simulink model "DroneControl_2018a"  (R2018a)
settings: Solver=VariableStepAuto  StartTime=0.0  StopTime=Tfinal  RelTol=1e-3
values from neighbouring files (symbols this model uses):
  body_rate_0 = [0;0;0]    [SetDroneControl_copy.m]
  Euler_0 = [0;0;0]    [SetDroneControl_copy.m]
  g = [0;0;-9.8]    [SetDroneControl_copy.m]
  I = [[0.1,0,0];[0,0.1,0];[0,0,0.08]]    [SetDroneControl_copy.m]
  m = 0.2    [SetDroneControl_copy.m]
  surround_rate = 0    [SetDroneControl_copy.m]
  ts = 0.01    [SetDroneControl_copy.m]
  XYZ_0 = [1;2;0]    [SetDroneControl_copy.m]
undefined symbols (not defined in the file or in its folder): Xcmd, Ycmd
libraries: simulink x18, vrlib x2, simulink_extras x1
settings Model: NumberOfSteps=10  Creator=blaze8871  LastModifiedBy=blaze8871
settings DataIOCC: SaveTime=off  ReturnWorkspaceOutputs=on
settings SFSimCC: SimUseLocalCustomCode=on
settings RTWCC: RTWUseLocalCustomCode=on

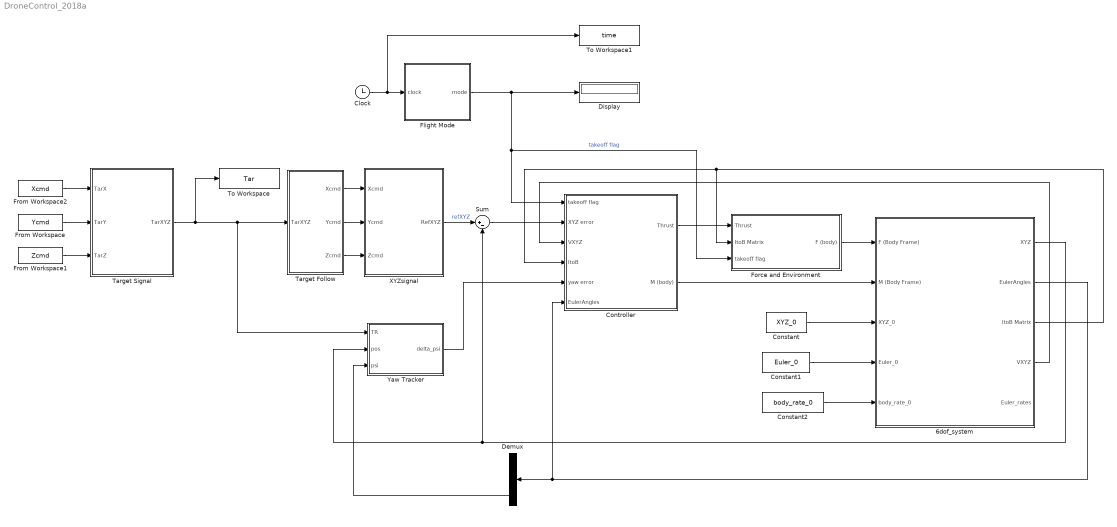
== system DroneControl_2018a ==
  6dof_system : Subsystem
  Clock : Clock
  Constant : Constant  Value=XYZ_0  SampleTime=0.01
  Constant1 : Constant  Value=Euler_0  SampleTime=0.01
  Constant2 : Constant  Value=body_rate_0  SampleTime=0.01
  Controller : Subsystem
  Demux : Demux  Outputs=3
  Display : Display
  Flight Mode : MATLAB Function  TreatAsAtomicUnit=on
  Force and Environment : Subsystem
  From Workspace : FromWorkspace  VariableName=Ycmd  SampleTime=ts
  From Workspace1 : FromWorkspace  VariableName=Zcmd  SampleTime=ts
  From Workspace2 : FromWorkspace  VariableName=Xcmd  SampleTime=ts
  Sum : Sum  Inputs=|+-
  Target Follow : Subsystem
  Target Signal : MATLAB Function  TreatAsAtomicUnit=on
  To Workspace : ToWorkspace  VariableName=Tar  SampleTime=ts
  To Workspace1 : ToWorkspace  VariableName=time  SampleTime=ts
  XYZsignal : MATLAB Function  TreatAsAtomicUnit=on
  Yaw Tracker : MATLAB Function  TreatAsAtomicUnit=on
  wires:
  Constant/1 -> 6dof_system/3(XYZ_0)
  Constant1/1 -> 6dof_system/4(Euler_0)
  Constant2/1 -> 6dof_system/5(body_rate_0)
  6dof_system/3(ItoB Matrix) -> Force and Environment/2(ItoB Matrix), Controller/4(ItoB)
  XYZsignal/1(RefXYZ) -> Sum/1  "refXYZ"
  6dof_system/1(XYZ) -> Sum/2, Yaw Tracker/2(pos)
  Clock/1 -> To Workspace1/1, Flight Mode/1(clock)
  Flight Mode/1(mode) -> Controller/1(takeoff flag), Force and Environment/3(takeoff flag), Display/1  "takeoff flag"
  Force and Environment/1(F (body)) -> 6dof_system/1(F (Body Frame))
  6dof_system/2(EulerAngles) -> Controller/6(EulerAngles), Demux/1
  Sum/1 -> Controller/2(XYZ error)
  6dof_system/4(VXYZ) -> Controller/3(VXYZ)
  Controller/2(M (body)) -> 6dof_system/2(M (Body Frame))
  Controller/1(Thrust) -> Force and Environment/1(Thrust)
  Demux/3 -> Yaw Tracker/3(psi)
  Yaw Tracker/1(delta_psi) -> Controller/5(yaw error)
  Target Signal/1(TarXYZ) -> To Workspace/1, Target Follow/1(TarXYZ), Yaw Tracker/1(TR)
  From Workspace2/1 -> Target Signal/1(TarX)
  From Workspace/1 -> Target Signal/2(TarY)
  From Workspace1/1 -> Target Signal/3(TarZ)
  Target Follow/1(Xcmd) -> XYZsignal/1(Xcmd)
  Target Follow/2(Ycmd) -> XYZsignal/2(Ycmd)
  Target Follow/3(Zcmd) -> XYZsignal/3(Zcmd)

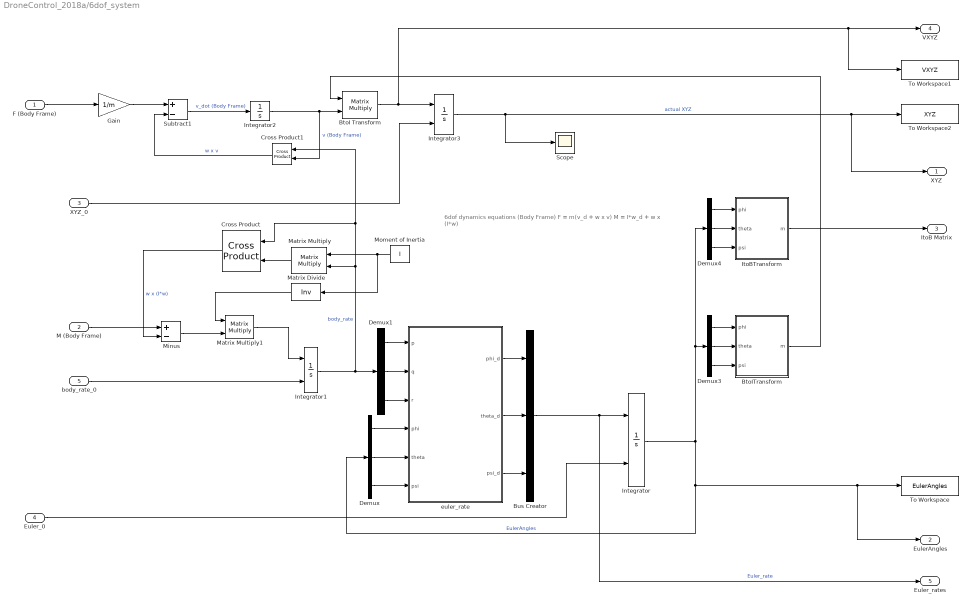
== system DroneControl_2018a/6dof_system ==
  note: 6dof dynamics equations
      | (Body Frame)
      |
      | F = m(v_d + w x v)
      | M = I*w_d + w x (I*w)
  F (Body Frame) : Inport
  M (Body Frame) : Inport  Port=2
  XYZ_0 : Inport  Port=3
  Euler_0 : Inport  Port=4
  body_rate_0 : Inport  Port=5
  BtoI Transform : Product  Multiplication=Matrix(*)
  BtoITransform : MATLAB Function  TreatAsAtomicUnit=on
  Bus Creator : BusCreator  Inputs=3
  Cross Product : vrlib/Utilities/Cross Product
  Cross Product1 : vrlib/Utilities/Cross Product
  Demux{,1,3..4} (4 alike) : Demux  Outputs=3
  Gain : Gain  Gain=1/m
  Integrator : Integrator  InitialConditionSource=external  ContinuousStateAttributes='EulerAngle'
  Integrator1 : Integrator  InitialConditionSource=external  ContinuousStateAttributes='EulerAngle'
  Integrator2 : Integrator
  Integrator3 : Integrator  InitialConditionSource=external
  ItoBTransform : MATLAB Function  TreatAsAtomicUnit=on
  Matrix Divide : Product  Inputs=/  Multiplication=Matrix(*)
  Matrix Multiply : Product  Multiplication=Matrix(*)
  Matrix Multiply1 : Product  Multiplication=Matrix(*)
  Minus : Sum  Inputs=+-
  Moment of Inertia : Constant  Value=I
  Scope : Scope
  Subtract1 : Sum  Inputs=+-
  To Workspace : ToWorkspace  VariableName=EulerAngles  SampleTime=ts
  To Workspace1 : ToWorkspace  VariableName=VXYZ  SampleTime=ts
  To Workspace2 : ToWorkspace  VariableName=XYZ  SampleTime=ts
  euler_rate : MATLAB Function  TreatAsAtomicUnit=on
  XYZ : Outport
  EulerAngles : Outport  Port=2
  ItoB Matrix : Outport  Port=3
  VXYZ : Outport  Port=4
  Euler_rates : Outport  Port=5
  wires:
  F (Body Frame)/1 -> Gain/1
  Demux4/2 -> ItoBTransform/2(theta)
  euler_rate/1(phi_d) -> Bus Creator/1
  BtoITransform/1(m) -> BtoI Transform/1
  Bus Creator/1 -> Euler_rates/1, Integrator/1  "Euler_rate"
  Matrix Multiply/1 -> Cross Product/2
  Moment of Inertia/1 -> Matrix Divide/1, Matrix Multiply/1
  Demux3/2 -> BtoITransform/2(theta)
  Demux/2 -> euler_rate/5(theta)
  Demux4/1 -> ItoBTransform/1(phi)
  Subtract1/1 -> Integrator2/1  "v_dot (Body Frame)"
  Cross Product1/1 -> Subtract1/2  "w x v"
  Demux1/1 -> euler_rate/1(p)
  Demux/3 -> euler_rate/6(psi)
  euler_rate/2(theta_d) -> Bus Creator/2
  Euler_0/1 -> Integrator/2
  Integrator3/1 -> XYZ/1, To Workspace2/1, Scope/1  "actual XYZ"
  Cross Product/1 -> Minus/2  "w x (I*w)"
  M (Body Frame)/1 -> Minus/1
  body_rate_0/1 -> Integrator1/2
  Demux3/3 -> BtoITransform/3(psi)
  euler_rate/3(psi_d) -> Bus Creator/3
  Demux4/3 -> ItoBTransform/3(psi)
  Gain/1 -> Subtract1/1
  Demux3/1 -> BtoITransform/1(phi)
  Demux1/3 -> euler_rate/3(r)
  XYZ_0/1 -> Integrator3/2
  Integrator/1 -> EulerAngles/1, To Workspace/1, Demux/1, Demux4/1, Demux3/1  "EulerAngles"
  Demux/1 -> euler_rate/4(phi)
  Integrator2/1 -> BtoI Transform/2, Cross Product1/2  "v (Body Frame)"
  Integrator1/1 -> Cross Product1/1, Cross Product/1, Matrix Multiply/2, Demux1/1  "body_rate"
  Demux1/2 -> euler_rate/2(q)
  ItoBTransform/1(m) -> ItoB Matrix/1
  BtoI Transform/1 -> To Workspace1/1, VXYZ/1, Integrator3/1
  Minus/1 -> Matrix Multiply1/2
  Matrix Multiply1/1 -> Integrator1/1
  Matrix Divide/1 -> Matrix Multiply1/1

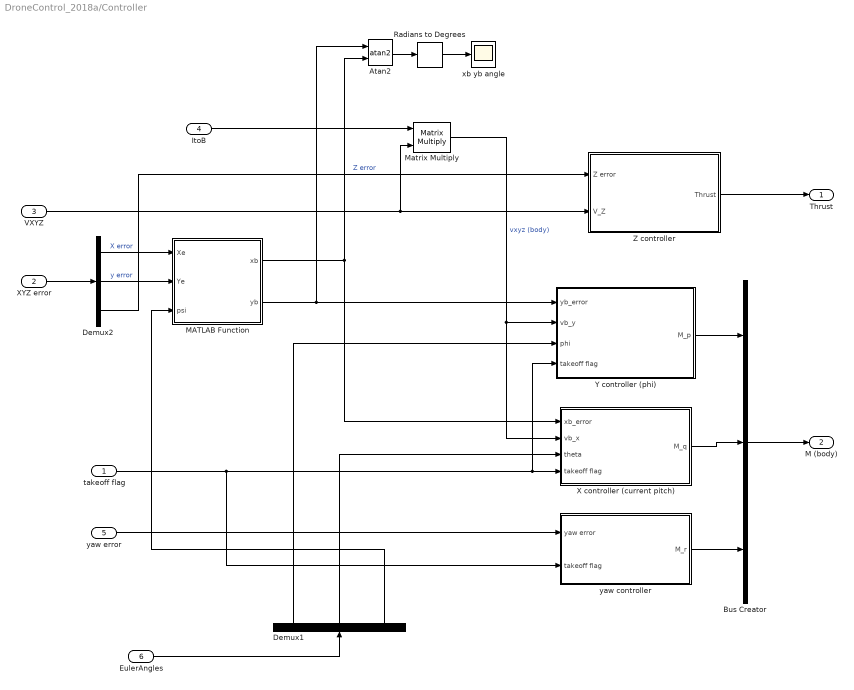
== system DroneControl_2018a/Controller ==
  takeoff flag : Inport
  XYZ error : Inport  Port=2
  VXYZ : Inport  Port=3
  ItoB : Inport  Port=4
  yaw error : Inport  Port=5
  EulerAngles : Inport  Port=6
  Atan2 : Trigonometry  Operator=atan2
  Bus Creator : BusCreator  Inputs=3
  Demux1 : Demux  Outputs=3
  Demux2 : Demux  Outputs=3
  MATLAB Function : MATLAB Function  TreatAsAtomicUnit=on
  Matrix Multiply : Product  Multiplication=Matrix(*)
  Radians to Degrees : simulink_extras/Transformations/Radians to Degrees
  X controller (current pitch) : Subsystem
  Y controller (phi) : Subsystem
  Z controller : Subsystem
  xb yb angle : Scope
  "yaw controller " : Subsystem
  Thrust : Outport
  M (body) : Outport  Port=2
  wires:
  Bus Creator/1 -> M (body)/1
  VXYZ/1 -> Z controller/2(V_Z), Matrix Multiply/2
  "yaw controller "/1(M_r) -> Bus Creator/3
  XYZ error/1 -> Demux2/1
  Demux1/1 -> Y controller (phi)/3(phi)
  Demux1/2 -> X controller (current pitch)/3(theta)
  Demux2/3 -> Z controller/1(Z error)  "Z error"
  takeoff flag/1 -> Y controller (phi)/4(takeoff flag), X controller (current pitch)/4(takeoff flag), "yaw controller "/2(takeoff flag)
  EulerAngles/1 -> Demux1/1
  Y controller (phi)/1(M_p) -> Bus Creator/1
  Demux1/3 -> MATLAB Function/3(psi)
  Z controller/1(Thrust) -> Thrust/1
  Demux2/2 -> MATLAB Function/2(Ye)  "y error"
  yaw error/1 -> "yaw controller "/1(yaw error)
  Demux2/1 -> MATLAB Function/1(Xe)  "X error"
  X controller (current pitch)/1(M_q) -> Bus Creator/2
  MATLAB Function/1(xb) -> X controller (current pitch)/1("xb_error "), Atan2/2
  MATLAB Function/2(yb) -> Atan2/1, Y controller (phi)/1("yb_error ")
  Atan2/1 -> Radians to Degrees/1
  Radians to Degrees/1 -> xb yb angle/1
  ItoB/1 -> Matrix Multiply/1
  Matrix Multiply/1 -> X controller (current pitch)/2(vb_x), Y controller (phi)/2(vb_y)  "vxyz (body)"

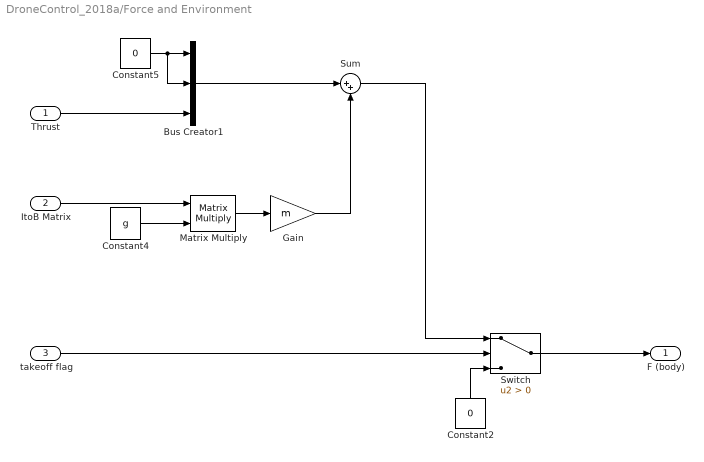
== system DroneControl_2018a/Force and Environment ==
  Thrust : Inport
  ItoB Matrix : Inport  Port=2
  takeoff flag : Inport  Port=3
  Bus Creator1 : BusCreator  Inputs=3
  Constant2 : Constant  Value=0  SampleTime=0.01
  Constant4 : Constant  Value=g  SampleTime=0.01
  Constant5 : Constant  Value=0  SampleTime=0.01
  Gain : Gain  Gain=m
  Matrix Multiply : Product  Multiplication=Matrix(*)
  Sum : Sum  Inputs=|++
  Switch : Switch  Criteria=u2 > Threshold
  F (body) : Outport
  wires:
  Thrust/1 -> Bus Creator1/3
  Bus Creator1/1 -> Sum/1
  Constant4/1 -> Matrix Multiply/2
  ItoB Matrix/1 -> Matrix Multiply/1
  Constant5/1 -> Bus Creator1/2, Bus Creator1/1
  takeoff flag/1 -> Switch/2
  Constant2/1 -> Switch/3
  Matrix Multiply/1 -> Gain/1
  Sum/1 -> Switch/1
  Switch/1 -> F (body)/1
  Gain/1 -> Sum/2

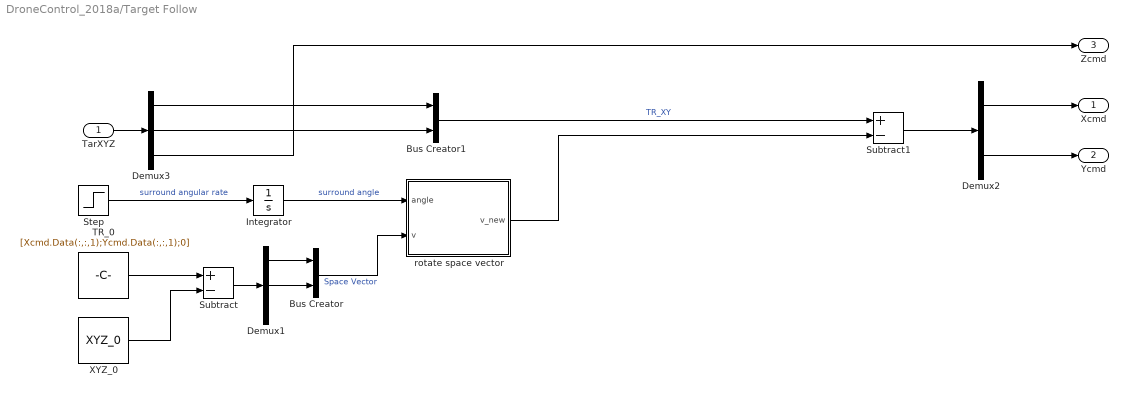
== system DroneControl_2018a/Target Follow ==
  TarXYZ : Inport
  Bus Creator : BusCreator  Inputs=2
  Bus Creator1 : BusCreator  Inputs=2
  Demux1 : Demux  Outputs=3
  Demux2 : Demux  Outputs=2
  Demux3 : Demux  Outputs=3
  Integrator : Integrator
  Step : Step  Time=2  After=surround_rate  SampleTime=0
  Subtract : Sum  Inputs=+-
  Subtract1 : Sum  Inputs=+-
  TR_0 : Constant  Value=[Xcmd.Data(:,:,1);Ycmd.Data(:,:,1);0]
  XYZ_0 : Constant  Value=XYZ_0
  rotate space vector : MATLAB Function  TreatAsAtomicUnit=on
  Xcmd : Outport
  Ycmd : Outport  Port=2
  Zcmd : Outport  Port=3
  wires:
  Subtract1/1 -> Demux2/1
  Demux2/2 -> Ycmd/1
  TR_0/1 -> Subtract/1
  Demux1/2 -> Bus Creator/2
  Bus Creator1/1 -> Subtract1/1  "TR_XY"
  TarXYZ/1 -> Demux3/1
  Demux3/2 -> Bus Creator1/2
  Subtract/1 -> Demux1/1
  Demux3/3 -> Zcmd/1
  Demux2/1 -> Xcmd/1
  Demux1/1 -> Bus Creator/1
  Demux3/1 -> Bus Creator1/1
  Bus Creator/1 -> rotate space vector/2(v)  "Space Vector"
  XYZ_0/1 -> Subtract/2
  Step/1 -> Integrator/1  "surround angular rate"
  Integrator/1 -> rotate space vector/1(angle)  "surround angle"
  rotate space vector/1(v_new) -> Subtract1/2

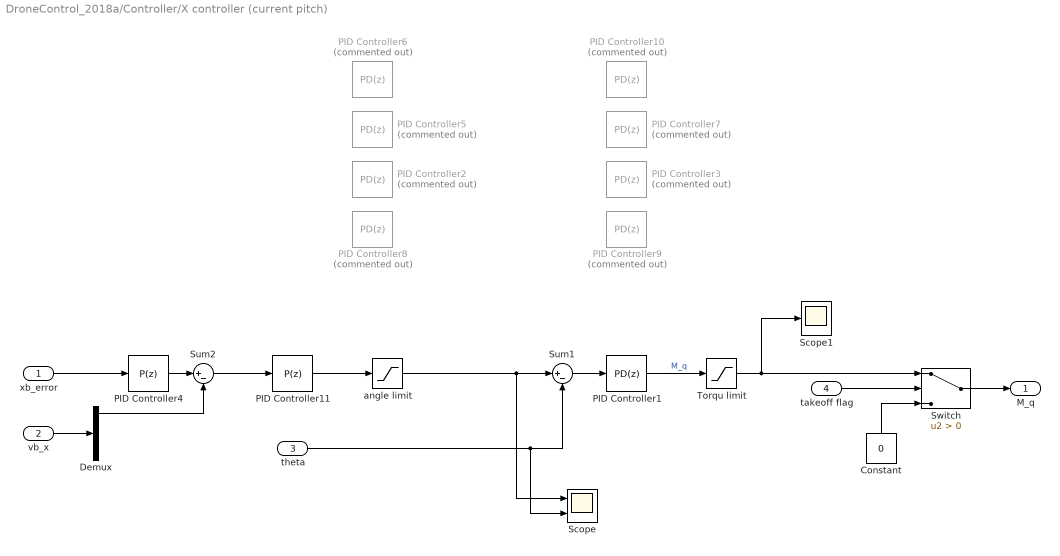
== system DroneControl_2018a/Controller/X controller (current pitch) ==
  "xb_error " : Inport
  vb_x : Inport  Port=2
  theta : Inport  Port=3
  takeoff flag : Inport  Port=4
  Constant : Constant  Value=0
  Demux : Demux  Outputs=3
  PID Controller1 : simulink/Continuous/PID Controller  Controller=PD  Form=Parallel  TimeDomain=Discrete-time  SampleTime=ts  IntegratorMethod=Forward Euler  FilterMethod=Forward Euler  ControllerParametersSource=internal  P=1.1  I=1  D=1.2  UseFilter=on  N=100  TunerSelectOption=Transfer Function Based (PID Tuner App)  InitialConditionSource=internal  InitialConditionForIntegrator=0  InitialConditionForFilter=0  DifferentiatorICPrevScaledInput=0  ExternalReset=none  TrackingMode=off  Kt=1  LimitOutput=off  UpperSaturationLimit=inf  LowerSaturationLimit=-inf  LinearizeAsGain=on  AntiWindupMode=none  Kb=1  POutMin=[]  POutMax=[]  IOutMin=[]  IOutMax=[]  DOutMin=[]  DOutMax=[]  NOutMin=[]  NOutMax=[]  SumOutMin=[]  SumOutMax=[]  SaturationOutMin=[]  SaturationOutMax=[]  PParamMin=[]  PParamMax=[]  IParamMin=[]  IParamMax=[]  DParamMin=[]  DParamMax=[]  NParamMin=[]  NParamMax=[]  KbParamMin=[]  KbParamMax=[]  KtParamMin=[]  KtParamMax=[]  KbOutMin=[]  KbOutMax=[]  KtOutMin=[]  KtOutMax=[]  IntegratorOutMin=[]  IntegratorOutMax=[]  FilterOutMin=[]  FilterOutMax=[]  SumI1OutMin=[]  SumI1OutMax=[]  SumI2OutMin=[]  SumI2OutMax=[]  SumI3OutMin=[]  SumI3OutMax=[]  SumDOutMin=[]  SumDOutMax=[]  DifferentiatorOutMin=[]  DifferentiatorOutMax=[]  FilterDiffOutCoefMin=[]  FilterDiffOutCoefMax=[]  ReciprocalOutMin=[]  ReciprocalOutMax=[]  SumDenOutMin=[]  SumDenOutMax=[]  SumNumOutMin=[]  SumNumOutMax=[]  DivideOutMin=[]  DivideOutMax=[]  IntegratorContinuousStateAttributes=''  IntegratorStateMustResolveToSignalObject=off  IntegratorRTWStateStorageClass=Auto  FilterContinuousStateAttributes=''  FilterStateMustResolveToSignalObject=off  FilterRTWStateStorageClass=Auto
  PID Controller10 : simulink/Continuous/PID Controller  Commented=on  Controller=PD  Form=Parallel  TimeDomain=Discrete-time  SampleTime=ts  IntegratorMethod=Forward Euler  FilterMethod=Forward Euler  ControllerParametersSource=internal  P=0.8  I=1  D=0.5  UseFilter=on  N=100  TunerSelectOption=Transfer Function Based (PID Tuner App)  InitialConditionSource=internal  InitialConditionForIntegrator=0  InitialConditionForFilter=0  DifferentiatorICPrevScaledInput=0  ExternalReset=none  TrackingMode=off  Kt=1  LimitOutput=off  UpperSaturationLimit=inf  LowerSaturationLimit=-inf  LinearizeAsGain=on  AntiWindupMode=none  Kb=1  POutMin=[]  POutMax=[]  IOutMin=[]  IOutMax=[]  DOutMin=[]  DOutMax=[]  NOutMin=[]  NOutMax=[]  SumOutMin=[]  SumOutMax=[]  SaturationOutMin=[]  SaturationOutMax=[]  PParamMin=[]  PParamMax=[]  IParamMin=[]  IParamMax=[]  DParamMin=[]  DParamMax=[]  NParamMin=[]  NParamMax=[]  KbParamMin=[]  KbParamMax=[]  KtParamMin=[]  KtParamMax=[]  KbOutMin=[]  KbOutMax=[]  KtOutMin=[]  KtOutMax=[]  IntegratorOutMin=[]  IntegratorOutMax=[]  FilterOutMin=[]  FilterOutMax=[]  SumI1OutMin=[]  SumI1OutMax=[]  SumI2OutMin=[]  SumI2OutMax=[]  SumI3OutMin=[]  SumI3OutMax=[]  SumDOutMin=[]  SumDOutMax=[]  DifferentiatorOutMin=[]  DifferentiatorOutMax=[]  FilterDiffOutCoefMin=[]  FilterDiffOutCoefMax=[]  ReciprocalOutMin=[]  ReciprocalOutMax=[]  SumDenOutMin=[]  SumDenOutMax=[]  SumNumOutMin=[]  SumNumOutMax=[]  DivideOutMin=[]  DivideOutMax=[]  IntegratorContinuousStateAttributes=''  IntegratorStateMustResolveToSignalObject=off  IntegratorRTWStateStorageClass=Auto  FilterContinuousStateAttributes=''  FilterStateMustResolveToSignalObject=off  FilterRTWStateStorageClass=Auto
  PID Controller11 : simulink/Continuous/PID Controller  Controller=P  Form=Parallel  TimeDomain=Discrete-time  SampleTime=ts  IntegratorMethod=Forward Euler  FilterMethod=Forward Euler  ControllerParametersSource=internal  P=0.2  I=1  D=0  UseFilter=on  N=100  TunerSelectOption=Transfer Function Based (PID Tuner App)  InitialConditionSource=internal  InitialConditionForIntegrator=0  InitialConditionForFilter=0  DifferentiatorICPrevScaledInput=0  ExternalReset=none  TrackingMode=off  Kt=1  LimitOutput=off  UpperSaturationLimit=inf  LowerSaturationLimit=-inf  LinearizeAsGain=on  AntiWindupMode=none  Kb=1  POutMin=[]  POutMax=[]  IOutMin=[]  IOutMax=[]  DOutMin=[]  DOutMax=[]  NOutMin=[]  NOutMax=[]  SumOutMin=[]  SumOutMax=[]  SaturationOutMin=[]  SaturationOutMax=[]  PParamMin=[]  PParamMax=[]  IParamMin=[]  IParamMax=[]  DParamMin=[]  DParamMax=[]  NParamMin=[]  NParamMax=[]  KbParamMin=[]  KbParamMax=[]  KtParamMin=[]  KtParamMax=[]  KbOutMin=[]  KbOutMax=[]  KtOutMin=[]  KtOutMax=[]  IntegratorOutMin=[]  IntegratorOutMax=[]  FilterOutMin=[]  FilterOutMax=[]  SumI1OutMin=[]  SumI1OutMax=[]  SumI2OutMin=[]  SumI2OutMax=[]  SumI3OutMin=[]  SumI3OutMax=[]  SumDOutMin=[]  SumDOutMax=[]  DifferentiatorOutMin=[]  DifferentiatorOutMax=[]  FilterDiffOutCoefMin=[]  FilterDiffOutCoefMax=[]  ReciprocalOutMin=[]  ReciprocalOutMax=[]  SumDenOutMin=[]  SumDenOutMax=[]  SumNumOutMin=[]  SumNumOutMax=[]  DivideOutMin=[]  DivideOutMax=[]  IntegratorContinuousStateAttributes=''  IntegratorStateMustResolveToSignalObject=off  IntegratorRTWStateStorageClass=Auto  FilterContinuousStateAttributes=''  FilterStateMustResolveToSignalObject=off  FilterRTWStateStorageClass=Auto
  PID Controller2 : simulink/Continuous/PID Controller  Commented=on  Controller=PD  Form=Parallel  TimeDomain=Discrete-time  SampleTime=ts  IntegratorMethod=Forward Euler  FilterMethod=Forward Euler  ControllerParametersSource=internal  P=0.5  I=0  D=0.2  UseFilter=on  N=10  TunerSelectOption=Transfer Function Based (PID Tuner App)  InitialConditionSource=internal  InitialConditionForIntegrator=0  InitialConditionForFilter=0  DifferentiatorICPrevScaledInput=0  ExternalReset=none  TrackingMode=off  Kt=1  LimitOutput=off  UpperSaturationLimit=inf  LowerSaturationLimit=-inf  LinearizeAsGain=on  AntiWindupMode=none  Kb=1  POutMin=[]  POutMax=[]  IOutMin=[]  IOutMax=[]  DOutMin=[]  DOutMax=[]  NOutMin=[]  NOutMax=[]  SumOutMin=[]  SumOutMax=[]  SaturationOutMin=[]  SaturationOutMax=[]  PParamMin=[]  PParamMax=[]  IParamMin=[]  IParamMax=[]  DParamMin=[]  DParamMax=[]  NParamMin=[]  NParamMax=[]  KbParamMin=[]  KbParamMax=[]  KtParamMin=[]  KtParamMax=[]  KbOutMin=[]  KbOutMax=[]  KtOutMin=[]  KtOutMax=[]  IntegratorOutMin=[]  IntegratorOutMax=[]  FilterOutMin=[]  FilterOutMax=[]  SumI1OutMin=[]  SumI1OutMax=[]  SumI2OutMin=[]  SumI2OutMax=[]  SumI3OutMin=[]  SumI3OutMax=[]  SumDOutMin=[]  SumDOutMax=[]  DifferentiatorOutMin=[]  DifferentiatorOutMax=[]  FilterDiffOutCoefMin=[]  FilterDiffOutCoefMax=[]  ReciprocalOutMin=[]  ReciprocalOutMax=[]  SumDenOutMin=[]  SumDenOutMax=[]  SumNumOutMin=[]  SumNumOutMax=[]  DivideOutMin=[]  DivideOutMax=[]  IntegratorContinuousStateAttributes=''  IntegratorStateMustResolveToSignalObject=off  IntegratorRTWStateStorageClass=Auto  FilterContinuousStateAttributes=''  FilterStateMustResolveToSignalObject=off  FilterRTWStateStorageClass=Auto
  PID Controller3 : simulink/Continuous/PID Controller  Commented=on  Controller=PD  Form=Parallel  TimeDomain=Discrete-time  SampleTime=ts  IntegratorMethod=Forward Euler  FilterMethod=Forward Euler  ControllerParametersSource=internal  P=1.5  I=1  D=2  UseFilter=on  N=100  TunerSelectOption=Transfer Function Based (PID Tuner App)  InitialConditionSource=internal  InitialConditionForIntegrator=0  InitialConditionForFilter=0  DifferentiatorICPrevScaledInput=0  ExternalReset=none  TrackingMode=off  Kt=1  LimitOutput=off  UpperSaturationLimit=inf  LowerSaturationLimit=-inf  LinearizeAsGain=on  AntiWindupMode=none  Kb=1  POutMin=[]  POutMax=[]  IOutMin=[]  IOutMax=[]  DOutMin=[]  DOutMax=[]  NOutMin=[]  NOutMax=[]  SumOutMin=[]  SumOutMax=[]  SaturationOutMin=[]  SaturationOutMax=[]  PParamMin=[]  PParamMax=[]  IParamMin=[]  IParamMax=[]  DParamMin=[]  DParamMax=[]  NParamMin=[]  NParamMax=[]  KbParamMin=[]  KbParamMax=[]  KtParamMin=[]  KtParamMax=[]  KbOutMin=[]  KbOutMax=[]  KtOutMin=[]  KtOutMax=[]  IntegratorOutMin=[]  IntegratorOutMax=[]  FilterOutMin=[]  FilterOutMax=[]  SumI1OutMin=[]  SumI1OutMax=[]  SumI2OutMin=[]  SumI2OutMax=[]  SumI3OutMin=[]  SumI3OutMax=[]  SumDOutMin=[]  SumDOutMax=[]  DifferentiatorOutMin=[]  DifferentiatorOutMax=[]  FilterDiffOutCoefMin=[]  FilterDiffOutCoefMax=[]  ReciprocalOutMin=[]  ReciprocalOutMax=[]  SumDenOutMin=[]  SumDenOutMax=[]  SumNumOutMin=[]  SumNumOutMax=[]  DivideOutMin=[]  DivideOutMax=[]  IntegratorContinuousStateAttributes=''  IntegratorStateMustResolveToSignalObject=off  IntegratorRTWStateStorageClass=Auto  FilterContinuousStateAttributes=''  FilterStateMustResolveToSignalObject=off  FilterRTWStateStorageClass=Auto
  PID Controller4 : simulink/Continuous/PID Controller  Controller=P  Form=Parallel  TimeDomain=Discrete-time  SampleTime=ts  IntegratorMethod=Forward Euler  FilterMethod=Forward Euler  ControllerParametersSource=internal  P=1.0  I=1  D=0  UseFilter=on  N=100  TunerSelectOption=Transfer Function Based (PID Tuner App)  InitialConditionSource=internal  InitialConditionForIntegrator=0  InitialConditionForFilter=0  DifferentiatorICPrevScaledInput=0  ExternalReset=none  TrackingMode=off  Kt=1  LimitOutput=off  UpperSaturationLimit=inf  LowerSaturationLimit=-inf  LinearizeAsGain=on  AntiWindupMode=none  Kb=1  POutMin=[]  POutMax=[]  IOutMin=[]  IOutMax=[]  DOutMin=[]  DOutMax=[]  NOutMin=[]  NOutMax=[]  SumOutMin=[]  SumOutMax=[]  SaturationOutMin=[]  SaturationOutMax=[]  PParamMin=[]  PParamMax=[]  IParamMin=[]  IParamMax=[]  DParamMin=[]  DParamMax=[]  NParamMin=[]  NParamMax=[]  KbParamMin=[]  KbParamMax=[]  KtParamMin=[]  KtParamMax=[]  KbOutMin=[]  KbOutMax=[]  KtOutMin=[]  KtOutMax=[]  IntegratorOutMin=[]  IntegratorOutMax=[]  FilterOutMin=[]  FilterOutMax=[]  SumI1OutMin=[]  SumI1OutMax=[]  SumI2OutMin=[]  SumI2OutMax=[]  SumI3OutMin=[]  SumI3OutMax=[]  SumDOutMin=[]  SumDOutMax=[]  DifferentiatorOutMin=[]  DifferentiatorOutMax=[]  FilterDiffOutCoefMin=[]  FilterDiffOutCoefMax=[]  ReciprocalOutMin=[]  ReciprocalOutMax=[]  SumDenOutMin=[]  SumDenOutMax=[]  SumNumOutMin=[]  SumNumOutMax=[]  DivideOutMin=[]  DivideOutMax=[]  IntegratorContinuousStateAttributes=''  IntegratorStateMustResolveToSignalObject=off  IntegratorRTWStateStorageClass=Auto  FilterContinuousStateAttributes=''  FilterStateMustResolveToSignalObject=off  FilterRTWStateStorageClass=Auto
  PID Controller5 : simulink/Continuous/PID Controller  Commented=on  Controller=PD  Form=Parallel  TimeDomain=Discrete-time  SampleTime=ts  IntegratorMethod=Forward Euler  FilterMethod=Forward Euler  ControllerParametersSource=internal  P=0.03  I=0  D=0.075  UseFilter=on  N=10  TunerSelectOption=Transfer Function Based (PID Tuner App)  InitialConditionSource=internal  InitialConditionForIntegrator=0  InitialConditionForFilter=0  DifferentiatorICPrevScaledInput=0  ExternalReset=none  TrackingMode=off  Kt=1  LimitOutput=off  UpperSaturationLimit=inf  LowerSaturationLimit=-inf  LinearizeAsGain=on  AntiWindupMode=none  Kb=1  POutMin=[]  POutMax=[]  IOutMin=[]  IOutMax=[]  DOutMin=[]  DOutMax=[]  NOutMin=[]  NOutMax=[]  SumOutMin=[]  SumOutMax=[]  SaturationOutMin=[]  SaturationOutMax=[]  PParamMin=[]  PParamMax=[]  IParamMin=[]  IParamMax=[]  DParamMin=[]  DParamMax=[]  NParamMin=[]  NParamMax=[]  KbParamMin=[]  KbParamMax=[]  KtParamMin=[]  KtParamMax=[]  KbOutMin=[]  KbOutMax=[]  KtOutMin=[]  KtOutMax=[]  IntegratorOutMin=[]  IntegratorOutMax=[]  FilterOutMin=[]  FilterOutMax=[]  SumI1OutMin=[]  SumI1OutMax=[]  SumI2OutMin=[]  SumI2OutMax=[]  SumI3OutMin=[]  SumI3OutMax=[]  SumDOutMin=[]  SumDOutMax=[]  DifferentiatorOutMin=[]  DifferentiatorOutMax=[]  FilterDiffOutCoefMin=[]  FilterDiffOutCoefMax=[]  ReciprocalOutMin=[]  ReciprocalOutMax=[]  SumDenOutMin=[]  SumDenOutMax=[]  SumNumOutMin=[]  SumNumOutMax=[]  DivideOutMin=[]  DivideOutMax=[]  IntegratorContinuousStateAttributes=''  IntegratorStateMustResolveToSignalObject=off  IntegratorRTWStateStorageClass=Auto  FilterContinuousStateAttributes=''  FilterStateMustResolveToSignalObject=off  FilterRTWStateStorageClass=Auto
  PID Controller6 : simulink/Continuous/PID Controller  Commented=on  Controller=PD  Form=Parallel  TimeDomain=Discrete-time  SampleTime=ts  IntegratorMethod=Forward Euler  FilterMethod=Forward Euler  ControllerParametersSource=internal  P=0.8  I=0  D=0.45  UseFilter=on  N=10  TunerSelectOption=Transfer Function Based (PID Tuner App)  InitialConditionSource=internal  InitialConditionForIntegrator=0  InitialConditionForFilter=0  DifferentiatorICPrevScaledInput=0  ExternalReset=none  TrackingMode=off  Kt=1  LimitOutput=off  UpperSaturationLimit=inf  LowerSaturationLimit=-inf  LinearizeAsGain=on  AntiWindupMode=none  Kb=1  POutMin=[]  POutMax=[]  IOutMin=[]  IOutMax=[]  DOutMin=[]  DOutMax=[]  NOutMin=[]  NOutMax=[]  SumOutMin=[]  SumOutMax=[]  SaturationOutMin=[]  SaturationOutMax=[]  PParamMin=[]  PParamMax=[]  IParamMin=[]  IParamMax=[]  DParamMin=[]  DParamMax=[]  NParamMin=[]  NParamMax=[]  KbParamMin=[]  KbParamMax=[]  KtParamMin=[]  KtParamMax=[]  KbOutMin=[]  KbOutMax=[]  KtOutMin=[]  KtOutMax=[]  IntegratorOutMin=[]  IntegratorOutMax=[]  FilterOutMin=[]  FilterOutMax=[]  SumI1OutMin=[]  SumI1OutMax=[]  SumI2OutMin=[]  SumI2OutMax=[]  SumI3OutMin=[]  SumI3OutMax=[]  SumDOutMin=[]  SumDOutMax=[]  DifferentiatorOutMin=[]  DifferentiatorOutMax=[]  FilterDiffOutCoefMin=[]  FilterDiffOutCoefMax=[]  ReciprocalOutMin=[]  ReciprocalOutMax=[]  SumDenOutMin=[]  SumDenOutMax=[]  SumNumOutMin=[]  SumNumOutMax=[]  DivideOutMin=[]  DivideOutMax=[]  IntegratorContinuousStateAttributes=''  IntegratorStateMustResolveToSignalObject=off  IntegratorRTWStateStorageClass=Auto  FilterContinuousStateAttributes=''  FilterStateMustResolveToSignalObject=off  FilterRTWStateStorageClass=Auto
  PID Controller7 : simulink/Continuous/PID Controller  Commented=on  Controller=PD  Form=Parallel  TimeDomain=Discrete-time  SampleTime=ts  IntegratorMethod=Forward Euler  FilterMethod=Forward Euler  ControllerParametersSource=internal  P=1.5  I=1  D=3.0  UseFilter=on  N=100  TunerSelectOption=Transfer Function Based (PID Tuner App)  InitialConditionSource=internal  InitialConditionForIntegrator=0  InitialConditionForFilter=0  DifferentiatorICPrevScaledInput=0  ExternalReset=none  TrackingMode=off  Kt=1  LimitOutput=off  UpperSaturationLimit=inf  LowerSaturationLimit=-inf  LinearizeAsGain=on  AntiWindupMode=none  Kb=1  POutMin=[]  POutMax=[]  IOutMin=[]  IOutMax=[]  DOutMin=[]  DOutMax=[]  NOutMin=[]  NOutMax=[]  SumOutMin=[]  SumOutMax=[]  SaturationOutMin=[]  SaturationOutMax=[]  PParamMin=[]  PParamMax=[]  IParamMin=[]  IParamMax=[]  DParamMin=[]  DParamMax=[]  NParamMin=[]  NParamMax=[]  KbParamMin=[]  KbParamMax=[]  KtParamMin=[]  KtParamMax=[]  KbOutMin=[]  KbOutMax=[]  KtOutMin=[]  KtOutMax=[]  IntegratorOutMin=[]  IntegratorOutMax=[]  FilterOutMin=[]  FilterOutMax=[]  SumI1OutMin=[]  SumI1OutMax=[]  SumI2OutMin=[]  SumI2OutMax=[]  SumI3OutMin=[]  SumI3OutMax=[]  SumDOutMin=[]  SumDOutMax=[]  DifferentiatorOutMin=[]  DifferentiatorOutMax=[]  FilterDiffOutCoefMin=[]  FilterDiffOutCoefMax=[]  ReciprocalOutMin=[]  ReciprocalOutMax=[]  SumDenOutMin=[]  SumDenOutMax=[]  SumNumOutMin=[]  SumNumOutMax=[]  DivideOutMin=[]  DivideOutMax=[]  IntegratorContinuousStateAttributes=''  IntegratorStateMustResolveToSignalObject=off  IntegratorRTWStateStorageClass=Auto  FilterContinuousStateAttributes=''  FilterStateMustResolveToSignalObject=off  FilterRTWStateStorageClass=Auto
  PID Controller8 : simulink/Continuous/PID Controller  Commented=on  Controller=PD  Form=Parallel  TimeDomain=Discrete-time  SampleTime=ts  IntegratorMethod=Forward Euler  FilterMethod=Forward Euler  ControllerParametersSource=internal  P=0.2  I=0  D=0.25  UseFilter=on  N=10  TunerSelectOption=Transfer Function Based (PID Tuner App)  InitialConditionSource=internal  InitialConditionForIntegrator=0  InitialConditionForFilter=0  DifferentiatorICPrevScaledInput=0  ExternalReset=none  TrackingMode=off  Kt=1  LimitOutput=off  UpperSaturationLimit=inf  LowerSaturationLimit=-inf  LinearizeAsGain=on  AntiWindupMode=none  Kb=1  POutMin=[]  POutMax=[]  IOutMin=[]  IOutMax=[]  DOutMin=[]  DOutMax=[]  NOutMin=[]  NOutMax=[]  SumOutMin=[]  SumOutMax=[]  SaturationOutMin=[]  SaturationOutMax=[]  PParamMin=[]  PParamMax=[]  IParamMin=[]  IParamMax=[]  DParamMin=[]  DParamMax=[]  NParamMin=[]  NParamMax=[]  KbParamMin=[]  KbParamMax=[]  KtParamMin=[]  KtParamMax=[]  KbOutMin=[]  KbOutMax=[]  KtOutMin=[]  KtOutMax=[]  IntegratorOutMin=[]  IntegratorOutMax=[]  FilterOutMin=[]  FilterOutMax=[]  SumI1OutMin=[]  SumI1OutMax=[]  SumI2OutMin=[]  SumI2OutMax=[]  SumI3OutMin=[]  SumI3OutMax=[]  SumDOutMin=[]  SumDOutMax=[]  DifferentiatorOutMin=[]  DifferentiatorOutMax=[]  FilterDiffOutCoefMin=[]  FilterDiffOutCoefMax=[]  ReciprocalOutMin=[]  ReciprocalOutMax=[]  SumDenOutMin=[]  SumDenOutMax=[]  SumNumOutMin=[]  SumNumOutMax=[]  DivideOutMin=[]  DivideOutMax=[]  IntegratorContinuousStateAttributes=''  IntegratorStateMustResolveToSignalObject=off  IntegratorRTWStateStorageClass=Auto  FilterContinuousStateAttributes=''  FilterStateMustResolveToSignalObject=off  FilterRTWStateStorageClass=Auto
  PID Controller9 : simulink/Continuous/PID Controller  Commented=on  Controller=PD  Form=Parallel  TimeDomain=Discrete-time  SampleTime=ts  IntegratorMethod=Forward Euler  FilterMethod=Forward Euler  ControllerParametersSource=internal  P=1.1  I=1  D=1.2  UseFilter=on  N=100  TunerSelectOption=Transfer Function Based (PID Tuner App)  InitialConditionSource=internal  InitialConditionForIntegrator=0  InitialConditionForFilter=0  DifferentiatorICPrevScaledInput=0  ExternalReset=none  TrackingMode=off  Kt=1  LimitOutput=off  UpperSaturationLimit=inf  LowerSaturationLimit=-inf  LinearizeAsGain=on  AntiWindupMode=none  Kb=1  POutMin=[]  POutMax=[]  IOutMin=[]  IOutMax=[]  DOutMin=[]  DOutMax=[]  NOutMin=[]  NOutMax=[]  SumOutMin=[]  SumOutMax=[]  SaturationOutMin=[]  SaturationOutMax=[]  PParamMin=[]  PParamMax=[]  IParamMin=[]  IParamMax=[]  DParamMin=[]  DParamMax=[]  NParamMin=[]  NParamMax=[]  KbParamMin=[]  KbParamMax=[]  KtParamMin=[]  KtParamMax=[]  KbOutMin=[]  KbOutMax=[]  KtOutMin=[]  KtOutMax=[]  IntegratorOutMin=[]  IntegratorOutMax=[]  FilterOutMin=[]  FilterOutMax=[]  SumI1OutMin=[]  SumI1OutMax=[]  SumI2OutMin=[]  SumI2OutMax=[]  SumI3OutMin=[]  SumI3OutMax=[]  SumDOutMin=[]  SumDOutMax=[]  DifferentiatorOutMin=[]  DifferentiatorOutMax=[]  FilterDiffOutCoefMin=[]  FilterDiffOutCoefMax=[]  ReciprocalOutMin=[]  ReciprocalOutMax=[]  SumDenOutMin=[]  SumDenOutMax=[]  SumNumOutMin=[]  SumNumOutMax=[]  DivideOutMin=[]  DivideOutMax=[]  IntegratorContinuousStateAttributes=''  IntegratorStateMustResolveToSignalObject=off  IntegratorRTWStateStorageClass=Auto  FilterContinuousStateAttributes=''  FilterStateMustResolveToSignalObject=off  FilterRTWStateStorageClass=Auto
  Scope : Scope  NumInputPorts=2
  Scope1 : Scope
  Sum1 : Sum  Inputs=|+-
  Sum2 : Sum  Inputs=|+-
  Switch : Switch  Criteria=u2 > Threshold
  Torqu limit : Saturate  UpperLimit=2  LowerLimit=-2
  angle limit : Saturate  UpperLimit=1.05  LowerLimit=-1.05
  M_q : Outport
  wires:
  Constant/1 -> Switch/3
  Switch/1 -> M_q/1
  angle limit/1 -> Sum1/1, Scope/1
  Sum1/1 -> PID Controller1/1
  PID Controller1/1 -> Torqu limit/1  "M_q"
  Torqu limit/1 -> Switch/1, Scope1/1
  theta/1 -> Sum1/2, Scope/2
  takeoff flag/1 -> Switch/2
  "xb_error "/1 -> PID Controller4/1
  Sum2/1 -> PID Controller11/1
  vb_x/1 -> Demux/1
  PID Controller11/1 -> angle limit/1
  PID Controller4/1 -> Sum2/1
  Demux/1 -> Sum2/2

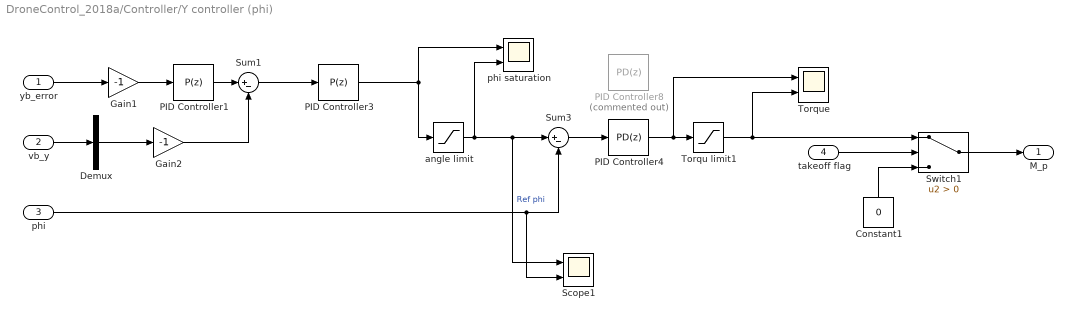
== system DroneControl_2018a/Controller/Y controller (phi) ==
  "yb_error " : Inport
  vb_y : Inport  Port=2
  phi : Inport  Port=3
  takeoff flag : Inport  Port=4
  " angle limit" : Saturate  UpperLimit=1.05  LowerLimit=-1.05
  Constant1 : Constant  Value=0
  Demux : Demux  Outputs=3
  Gain1 : Gain  Gain=-1
  Gain2 : Gain  Gain=-1
  PID Controller1 : simulink/Continuous/PID Controller  Controller=P  Form=Parallel  TimeDomain=Discrete-time  SampleTime=ts  IntegratorMethod=Forward Euler  FilterMethod=Forward Euler  ControllerParametersSource=internal  P=1.0  I=1  D=0  UseFilter=on  N=100  TunerSelectOption=Transfer Function Based (PID Tuner App)  InitialConditionSource=internal  InitialConditionForIntegrator=0  InitialConditionForFilter=0  DifferentiatorICPrevScaledInput=0  ExternalReset=none  TrackingMode=off  Kt=1  LimitOutput=off  UpperSaturationLimit=inf  LowerSaturationLimit=-inf  LinearizeAsGain=on  AntiWindupMode=none  Kb=1  POutMin=[]  POutMax=[]  IOutMin=[]  IOutMax=[]  DOutMin=[]  DOutMax=[]  NOutMin=[]  NOutMax=[]  SumOutMin=[]  SumOutMax=[]  SaturationOutMin=[]  SaturationOutMax=[]  PParamMin=[]  PParamMax=[]  IParamMin=[]  IParamMax=[]  DParamMin=[]  DParamMax=[]  NParamMin=[]  NParamMax=[]  KbParamMin=[]  KbParamMax=[]  KtParamMin=[]  KtParamMax=[]  KbOutMin=[]  KbOutMax=[]  KtOutMin=[]  KtOutMax=[]  IntegratorOutMin=[]  IntegratorOutMax=[]  FilterOutMin=[]  FilterOutMax=[]  SumI1OutMin=[]  SumI1OutMax=[]  SumI2OutMin=[]  SumI2OutMax=[]  SumI3OutMin=[]  SumI3OutMax=[]  SumDOutMin=[]  SumDOutMax=[]  DifferentiatorOutMin=[]  DifferentiatorOutMax=[]  FilterDiffOutCoefMin=[]  FilterDiffOutCoefMax=[]  ReciprocalOutMin=[]  ReciprocalOutMax=[]  SumDenOutMin=[]  SumDenOutMax=[]  SumNumOutMin=[]  SumNumOutMax=[]  DivideOutMin=[]  DivideOutMax=[]  IntegratorContinuousStateAttributes=''  IntegratorStateMustResolveToSignalObject=off  IntegratorRTWStateStorageClass=Auto  FilterContinuousStateAttributes=''  FilterStateMustResolveToSignalObject=off  FilterRTWStateStorageClass=Auto
  PID Controller3 : simulink/Continuous/PID Controller  Controller=P  Form=Parallel  TimeDomain=Discrete-time  SampleTime=ts  IntegratorMethod=Forward Euler  FilterMethod=Forward Euler  ControllerParametersSource=internal  P=0.2  I=1  D=0  UseFilter=on  N=100  TunerSelectOption=Transfer Function Based (PID Tuner App)  InitialConditionSource=internal  InitialConditionForIntegrator=0  InitialConditionForFilter=0  DifferentiatorICPrevScaledInput=0  ExternalReset=none  TrackingMode=off  Kt=1  LimitOutput=off  UpperSaturationLimit=inf  LowerSaturationLimit=-inf  LinearizeAsGain=on  AntiWindupMode=none  Kb=1  POutMin=[]  POutMax=[]  IOutMin=[]  IOutMax=[]  DOutMin=[]  DOutMax=[]  NOutMin=[]  NOutMax=[]  SumOutMin=[]  SumOutMax=[]  SaturationOutMin=[]  SaturationOutMax=[]  PParamMin=[]  PParamMax=[]  IParamMin=[]  IParamMax=[]  DParamMin=[]  DParamMax=[]  NParamMin=[]  NParamMax=[]  KbParamMin=[]  KbParamMax=[]  KtParamMin=[]  KtParamMax=[]  KbOutMin=[]  KbOutMax=[]  KtOutMin=[]  KtOutMax=[]  IntegratorOutMin=[]  IntegratorOutMax=[]  FilterOutMin=[]  FilterOutMax=[]  SumI1OutMin=[]  SumI1OutMax=[]  SumI2OutMin=[]  SumI2OutMax=[]  SumI3OutMin=[]  SumI3OutMax=[]  SumDOutMin=[]  SumDOutMax=[]  DifferentiatorOutMin=[]  DifferentiatorOutMax=[]  FilterDiffOutCoefMin=[]  FilterDiffOutCoefMax=[]  ReciprocalOutMin=[]  ReciprocalOutMax=[]  SumDenOutMin=[]  SumDenOutMax=[]  SumNumOutMin=[]  SumNumOutMax=[]  DivideOutMin=[]  DivideOutMax=[]  IntegratorContinuousStateAttributes=''  IntegratorStateMustResolveToSignalObject=off  IntegratorRTWStateStorageClass=Auto  FilterContinuousStateAttributes=''  FilterStateMustResolveToSignalObject=off  FilterRTWStateStorageClass=Auto
  PID Controller4 : simulink/Continuous/PID Controller  Controller=PD  Form=Parallel  TimeDomain=Discrete-time  SampleTime=ts  IntegratorMethod=Forward Euler  FilterMethod=Forward Euler  ControllerParametersSource=internal  P=1.1  I=0.05  D=0.45  UseFilter=on  N=60  TunerSelectOption=Transfer Function Based (PID Tuner App)  InitialConditionSource=internal  InitialConditionForIntegrator=0  InitialConditionForFilter=0  DifferentiatorICPrevScaledInput=0  ExternalReset=none  TrackingMode=off  Kt=1  LimitOutput=off  UpperSaturationLimit=inf  LowerSaturationLimit=-inf  LinearizeAsGain=on  AntiWindupMode=none  Kb=1  POutMin=[]  POutMax=[]  IOutMin=[]  IOutMax=[]  DOutMin=[]  DOutMax=[]  NOutMin=[]  NOutMax=[]  SumOutMin=[]  SumOutMax=[]  SaturationOutMin=[]  SaturationOutMax=[]  PParamMin=[]  PParamMax=[]  IParamMin=[]  IParamMax=[]  DParamMin=[]  DParamMax=[]  NParamMin=[]  NParamMax=[]  KbParamMin=[]  KbParamMax=[]  KtParamMin=[]  KtParamMax=[]  KbOutMin=[]  KbOutMax=[]  KtOutMin=[]  KtOutMax=[]  IntegratorOutMin=[]  IntegratorOutMax=[]  FilterOutMin=[]  FilterOutMax=[]  SumI1OutMin=[]  SumI1OutMax=[]  SumI2OutMin=[]  SumI2OutMax=[]  SumI3OutMin=[]  SumI3OutMax=[]  SumDOutMin=[]  SumDOutMax=[]  DifferentiatorOutMin=[]  DifferentiatorOutMax=[]  FilterDiffOutCoefMin=[]  FilterDiffOutCoefMax=[]  ReciprocalOutMin=[]  ReciprocalOutMax=[]  SumDenOutMin=[]  SumDenOutMax=[]  SumNumOutMin=[]  SumNumOutMax=[]  DivideOutMin=[]  DivideOutMax=[]  IntegratorContinuousStateAttributes=''  IntegratorStateMustResolveToSignalObject=off  IntegratorRTWStateStorageClass=Auto  FilterContinuousStateAttributes=''  FilterStateMustResolveToSignalObject=off  FilterRTWStateStorageClass=Auto
  PID Controller8 : simulink/Continuous/PID Controller  Commented=on  Controller=PD  Form=Parallel  TimeDomain=Discrete-time  SampleTime=ts  IntegratorMethod=Forward Euler  FilterMethod=Forward Euler  ControllerParametersSource=internal  P=1.1  I=0.05  D=0.45  UseFilter=on  N=100  TunerSelectOption=Transfer Function Based (PID Tuner App)  InitialConditionSource=internal  InitialConditionForIntegrator=0  InitialConditionForFilter=0  DifferentiatorICPrevScaledInput=0  ExternalReset=none  TrackingMode=off  Kt=1  LimitOutput=off  UpperSaturationLimit=inf  LowerSaturationLimit=-inf  LinearizeAsGain=on  AntiWindupMode=none  Kb=1  POutMin=[]  POutMax=[]  IOutMin=[]  IOutMax=[]  DOutMin=[]  DOutMax=[]  NOutMin=[]  NOutMax=[]  SumOutMin=[]  SumOutMax=[]  SaturationOutMin=[]  SaturationOutMax=[]  PParamMin=[]  PParamMax=[]  IParamMin=[]  IParamMax=[]  DParamMin=[]  DParamMax=[]  NParamMin=[]  NParamMax=[]  KbParamMin=[]  KbParamMax=[]  KtParamMin=[]  KtParamMax=[]  KbOutMin=[]  KbOutMax=[]  KtOutMin=[]  KtOutMax=[]  IntegratorOutMin=[]  IntegratorOutMax=[]  FilterOutMin=[]  FilterOutMax=[]  SumI1OutMin=[]  SumI1OutMax=[]  SumI2OutMin=[]  SumI2OutMax=[]  SumI3OutMin=[]  SumI3OutMax=[]  SumDOutMin=[]  SumDOutMax=[]  DifferentiatorOutMin=[]  DifferentiatorOutMax=[]  FilterDiffOutCoefMin=[]  FilterDiffOutCoefMax=[]  ReciprocalOutMin=[]  ReciprocalOutMax=[]  SumDenOutMin=[]  SumDenOutMax=[]  SumNumOutMin=[]  SumNumOutMax=[]  DivideOutMin=[]  DivideOutMax=[]  IntegratorContinuousStateAttributes=''  IntegratorStateMustResolveToSignalObject=off  IntegratorRTWStateStorageClass=Auto  FilterContinuousStateAttributes=''  FilterStateMustResolveToSignalObject=off  FilterRTWStateStorageClass=Auto
  Scope1 : Scope  NumInputPorts=2
  Sum1 : Sum  Inputs=|+-
  Sum3 : Sum  Inputs=|+-
  Switch1 : Switch  Criteria=u2 > Threshold
  Torqu limit1 : Saturate  UpperLimit=2  LowerLimit=-2
  Torque : Scope  NumInputPorts=2
  phi saturation : Scope  NumInputPorts=2
  M_p : Outport
  wires:
  PID Controller1/1 -> Sum1/1
  Sum1/1 -> PID Controller3/1
  vb_y/1 -> Demux/1
  Demux/2 -> Gain2/1
  Gain2/1 -> Sum1/2
  phi/1 -> Sum3/2, Scope1/2
  Sum3/1 -> PID Controller4/1
  takeoff flag/1 -> Switch1/2
  PID Controller4/1 -> Torque/1, Torqu limit1/1
  Switch1/1 -> M_p/1
  Gain1/1 -> PID Controller1/1
  Torqu limit1/1 -> Torque/2, Switch1/1
  " angle limit"/1 -> phi saturation/2, Sum3/1, Scope1/1  "Ref phi"
  Constant1/1 -> Switch1/3
  "yb_error "/1 -> Gain1/1
  PID Controller3/1 -> " angle limit"/1, phi saturation/1

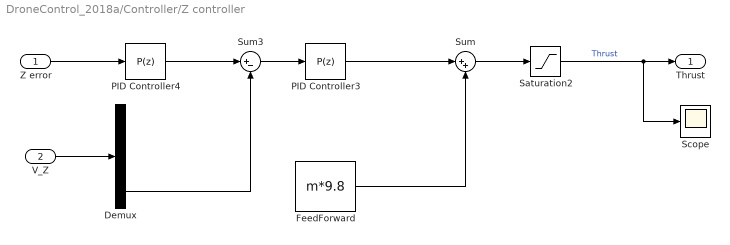
== system DroneControl_2018a/Controller/Z controller ==
  Z error : Inport
  V_Z : Inport  Port=2
  Demux : Demux  Outputs=3
  FeedForward : Constant  Value=m*9.8
  PID Controller3 : simulink/Continuous/PID Controller  Controller=P  Form=Parallel  TimeDomain=Discrete-time  SampleTime=ts  IntegratorMethod=Forward Euler  FilterMethod=Forward Euler  ControllerParametersSource=internal  P=1.51679141302942  I=1  D=0  UseFilter=on  N=100  TunerSelectOption=Transfer Function Based (PID Tuner App)  InitialConditionSource=internal  InitialConditionForIntegrator=0  InitialConditionForFilter=0  DifferentiatorICPrevScaledInput=0  ExternalReset=none  TrackingMode=off  Kt=1  LimitOutput=off  UpperSaturationLimit=inf  LowerSaturationLimit=-inf  LinearizeAsGain=on  AntiWindupMode=none  Kb=1  POutMin=[]  POutMax=[]  IOutMin=[]  IOutMax=[]  DOutMin=[]  DOutMax=[]  NOutMin=[]  NOutMax=[]  SumOutMin=[]  SumOutMax=[]  SaturationOutMin=[]  SaturationOutMax=[]  PParamMin=[]  PParamMax=[]  IParamMin=[]  IParamMax=[]  DParamMin=[]  DParamMax=[]  NParamMin=[]  NParamMax=[]  KbParamMin=[]  KbParamMax=[]  KtParamMin=[]  KtParamMax=[]  KbOutMin=[]  KbOutMax=[]  KtOutMin=[]  KtOutMax=[]  IntegratorOutMin=[]  IntegratorOutMax=[]  FilterOutMin=[]  FilterOutMax=[]  SumI1OutMin=[]  SumI1OutMax=[]  SumI2OutMin=[]  SumI2OutMax=[]  SumI3OutMin=[]  SumI3OutMax=[]  SumDOutMin=[]  SumDOutMax=[]  DifferentiatorOutMin=[]  DifferentiatorOutMax=[]  FilterDiffOutCoefMin=[]  FilterDiffOutCoefMax=[]  ReciprocalOutMin=[]  ReciprocalOutMax=[]  SumDenOutMin=[]  SumDenOutMax=[]  SumNumOutMin=[]  SumNumOutMax=[]  DivideOutMin=[]  DivideOutMax=[]  IntegratorContinuousStateAttributes=''  IntegratorStateMustResolveToSignalObject=off  IntegratorRTWStateStorageClass=Auto  FilterContinuousStateAttributes=''  FilterStateMustResolveToSignalObject=off  FilterRTWStateStorageClass=Auto
  PID Controller4 : simulink/Continuous/PID Controller  Controller=P  Form=Parallel  TimeDomain=Discrete-time  SampleTime=ts  IntegratorMethod=Forward Euler  FilterMethod=Forward Euler  ControllerParametersSource=internal  P=2.48254445381199  I=1  D=0  UseFilter=on  N=100  TunerSelectOption=Transfer Function Based (PID Tuner App)  InitialConditionSource=internal  InitialConditionForIntegrator=0  InitialConditionForFilter=0  DifferentiatorICPrevScaledInput=0  ExternalReset=none  TrackingMode=off  Kt=1  LimitOutput=off  UpperSaturationLimit=inf  LowerSaturationLimit=-inf  LinearizeAsGain=on  AntiWindupMode=none  Kb=1  POutMin=[]  POutMax=[]  IOutMin=[]  IOutMax=[]  DOutMin=[]  DOutMax=[]  NOutMin=[]  NOutMax=[]  SumOutMin=[]  SumOutMax=[]  SaturationOutMin=[]  SaturationOutMax=[]  PParamMin=[]  PParamMax=[]  IParamMin=[]  IParamMax=[]  DParamMin=[]  DParamMax=[]  NParamMin=[]  NParamMax=[]  KbParamMin=[]  KbParamMax=[]  KtParamMin=[]  KtParamMax=[]  KbOutMin=[]  KbOutMax=[]  KtOutMin=[]  KtOutMax=[]  IntegratorOutMin=[]  IntegratorOutMax=[]  FilterOutMin=[]  FilterOutMax=[]  SumI1OutMin=[]  SumI1OutMax=[]  SumI2OutMin=[]  SumI2OutMax=[]  SumI3OutMin=[]  SumI3OutMax=[]  SumDOutMin=[]  SumDOutMax=[]  DifferentiatorOutMin=[]  DifferentiatorOutMax=[]  FilterDiffOutCoefMin=[]  FilterDiffOutCoefMax=[]  ReciprocalOutMin=[]  ReciprocalOutMax=[]  SumDenOutMin=[]  SumDenOutMax=[]  SumNumOutMin=[]  SumNumOutMax=[]  DivideOutMin=[]  DivideOutMax=[]  IntegratorContinuousStateAttributes=''  IntegratorStateMustResolveToSignalObject=off  IntegratorRTWStateStorageClass=Auto  FilterContinuousStateAttributes=''  FilterStateMustResolveToSignalObject=off  FilterRTWStateStorageClass=Auto
  Saturation2 : Saturate  UpperLimit=30  LowerLimit=-30
  Scope : Scope
  Sum : Sum  Inputs=|++
  Sum3 : Sum  Inputs=|+-
  Thrust : Outport
  wires:
  V_Z/1 -> Demux/1
  PID Controller4/1 -> Sum3/1
  Sum3/1 -> PID Controller3/1
  Z error/1 -> PID Controller4/1
  Demux/3 -> Sum3/2
  PID Controller3/1 -> Sum/1
  Sum/1 -> Saturation2/1
  FeedForward/1 -> Sum/2
  Saturation2/1 -> Scope/1, Thrust/1  "Thrust"

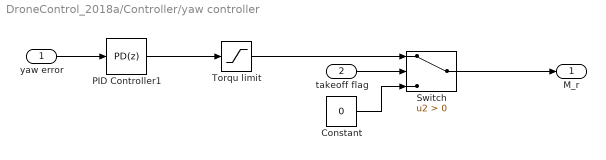
== system DroneControl_2018a/Controller/yaw controller  ==
  yaw error : Inport
  takeoff flag : Inport  Port=2
  Constant : Constant  Value=0
  PID Controller1 : simulink/Continuous/PID Controller  Controller=PD  Form=Parallel  TimeDomain=Discrete-time  SampleTime=ts  IntegratorMethod=Forward Euler  FilterMethod=Forward Euler  ControllerParametersSource=internal  P=0.6  I=1  D=0.4  UseFilter=on  N=10  TunerSelectOption=Transfer Function Based (PID Tuner App)  InitialConditionSource=internal  InitialConditionForIntegrator=0  InitialConditionForFilter=0  DifferentiatorICPrevScaledInput=0  ExternalReset=none  TrackingMode=off  Kt=1  LimitOutput=off  UpperSaturationLimit=inf  LowerSaturationLimit=-inf  LinearizeAsGain=on  AntiWindupMode=none  Kb=1  POutMin=[]  POutMax=[]  IOutMin=[]  IOutMax=[]  DOutMin=[]  DOutMax=[]  NOutMin=[]  NOutMax=[]  SumOutMin=[]  SumOutMax=[]  SaturationOutMin=[]  SaturationOutMax=[]  PParamMin=[]  PParamMax=[]  IParamMin=[]  IParamMax=[]  DParamMin=[]  DParamMax=[]  NParamMin=[]  NParamMax=[]  KbParamMin=[]  KbParamMax=[]  KtParamMin=[]  KtParamMax=[]  KbOutMin=[]  KbOutMax=[]  KtOutMin=[]  KtOutMax=[]  IntegratorOutMin=[]  IntegratorOutMax=[]  FilterOutMin=[]  FilterOutMax=[]  SumI1OutMin=[]  SumI1OutMax=[]  SumI2OutMin=[]  SumI2OutMax=[]  SumI3OutMin=[]  SumI3OutMax=[]  SumDOutMin=[]  SumDOutMax=[]  DifferentiatorOutMin=[]  DifferentiatorOutMax=[]  FilterDiffOutCoefMin=[]  FilterDiffOutCoefMax=[]  ReciprocalOutMin=[]  ReciprocalOutMax=[]  SumDenOutMin=[]  SumDenOutMax=[]  SumNumOutMin=[]  SumNumOutMax=[]  DivideOutMin=[]  DivideOutMax=[]  IntegratorContinuousStateAttributes=''  IntegratorStateMustResolveToSignalObject=off  IntegratorRTWStateStorageClass=Auto  FilterContinuousStateAttributes=''  FilterStateMustResolveToSignalObject=off  FilterRTWStateStorageClass=Auto
  Switch : Switch  Criteria=u2 > Threshold
  Torqu limit : Saturate  UpperLimit=1.5  LowerLimit=-1.5
  M_r : Outport
  wires:
  PID Controller1/1 -> Torqu limit/1
  yaw error/1 -> PID Controller1/1
  Switch/1 -> M_r/1
  Constant/1 -> Switch/3
  takeoff flag/1 -> Switch/2
  Torqu limit/1 -> Switch/1

== matlab function DroneControl_2018a/6dof_system/BtoITransform ==
  data: phi input; m output; theta input; psi input
function m = fcn(phi,theta,psi)
    T_BtoV2 = [[1 0 0];[0 cos(-phi) sin(-phi)];[0 -sin(-phi) cos(-phi)]];
    T_V2toV1 = [[cos(-theta) 0 -sin(-theta)];[0 1 0];[sin(-theta) 0 cos(-theta)]];
    T_V1toI = [[cos(-psi) sin(-psi) 0];[-sin(-psi) cos(-psi) 0];[0 0 1]];
    m = T_V1toI*T_V2toV1*T_BtoV2;

== matlab function DroneControl_2018a/6dof_system/euler_rate ==
  data: p input; phi_d output; q input; r input; phi input; theta input; theta_d output; psi_d output; psi input
function [phi_d,theta_d,psi_d] = fcn(p,q,r,phi,theta,psi)
    D = [[1 sin(phi)*tan(theta) cos(phi)*tan(theta)];
         [0 cos(phi) -sin(phi)];
         [0 sin(phi)/cos(theta) cos(phi)/cos(theta)]];
    euler_rate = D*[p;q;r]
    phi_d = euler_rate(1)
    theta_d = euler_rate(2)
    psi_d = euler_rate(3)

== matlab function DroneControl_2018a/Controller/MATLAB Function ==
  data: Xe input; xb output; Ye input; psi input; yb output
function [xb,yb] = fcn(Xe,Ye,psi)
    m = [[cos(psi) sin(psi)];[-sin(psi) cos(psi)]]
    pos = m*[Xe;Ye]
    xb = pos(1)
    yb = pos(2)

== matlab function DroneControl_2018a/XYZsignal ==
  data: Xcmd input; RefXYZ output; Ycmd input; Zcmd input
function RefXYZ = fcn(Xcmd,Ycmd,Zcmd)

RefXYZ = [Xcmd;Ycmd;Zcmd]

== matlab function DroneControl_2018a/6dof_system/ItoBTransform ==
  data: phi input; m output; theta input; psi input
function m = fcn(phi,theta,psi)
    T_ItoV1 = [[cos(psi) sin(psi) 0];[-sin(psi) cos(psi) 0];[0 0 1]]; 
    T_V1toV2 = [[cos(theta) 0 -sin(theta)];[0 1 0];[sin(theta) 0 cos(theta)]];
    T_V2toB = [[1 0 0];[0 cos(phi) sin(phi)];[0 -sin(phi) cos(phi)]];
    m = T_V2toB*T_V1toV2*T_ItoV1

== matlab function DroneControl_2018a/Yaw Tracker ==
  data: TR input; delta_psi output; pos input; psi input
function delta_psi = fcn(TR,pos,psi)
    v = [TR(1)-pos(1);TR(2)-pos(2)]
    v = v/norm(v)
    m = [[cos(psi) sin(psi)];[-sin(psi) cos(psi)]]
    v_b = m*v
    delta_psi = atan2(v_b(2),v_b(1))

== matlab function DroneControl_2018a/Flight Mode ==
  data: clock input; mode output
function mode = fcn(clock)
if clock <= 1
    mode = 0
elseif clock <= 3
    mode = 1
else
    mode = 2    
end

== matlab function DroneControl_2018a/Target Follow/rotate space vector ==
  data: angle input; v_new output; v input
function v_new = fcn(angle,v)
    m = [[cos(angle) -sin(angle)];[sin(angle) cos(angle)]]
    v_new = m*v

== matlab function DroneControl_2018a/Target Signal ==
  data: TarX input; TarXYZ output; TarY input; TarZ input
function TarXYZ = fcn(TarX,TarY,TarZ)

TarXYZ = [TarX;TarY;TarZ]
